simulink library "GTM_aerolib"  (Simulink 7.2)
settings: Solver=ode45  SolverMode=SingleTasking  StartTime=0.0  StopTime=10.0  RelTol=1e-3
undefined symbols (not defined in the file or in its folder): Aero, DamageModels
libraries: simulink_need_slupdate x58, GTM_aerolib x8, simulink x3
(part 2 of 3)

== system GTM_aerolib/Merged Control Surfaces/Spoilers ==
  alpha : Inport  OutDataType=sfix(16)  OutScaling=2^0
  beta : Inport  Port=2  OutDataType=sfix(16)  OutScaling=2^0
  Left : Inport  Port=3  OutDataType=sfix(16)  OutScaling=2^0
  Right : Inport  Port=4  OutDataType=sfix(16)  OutScaling=2^0
  Constant1 : Constant  Value=[0:5]  OutDataTypeMode=uint32  OutDataType=sfix(16)  OutScaling=2^0  OutDataTypeStr=uint32
  Constant2 : Constant  Value=[0:5]  OutDataTypeMode=uint32  OutDataType=sfix(16)  OutScaling=2^0  OutDataTypeStr=uint32
  Gain2 : Gain  Gain=-1  ParameterDataType=sfix(16)  ParameterScaling=2^0  OutDataType=sfix(16)  OutScaling=2^0
  Negate Lateral : Gain  Gain=[1 -1 1 -1 1 -1]  ParameterDataType=sfix(16)  ParameterScaling=2^0  OutDataType=sfix(16)  OutScaling=2^0
  PreLookup Index Search : simulink_need_slupdate/PreLookup Index Search  bpData=Aero.dC6_spo.alpha  searchMode=Binary Search  cacheBpFlag=on  outputFlag=off  IndexDataType=uint32  extrapMode=Linear Extrapolation  rangeErrorMode=None
  PreLookup Index Search1 : simulink_need_slupdate/PreLookup Index Search  bpData=Aero.dC6_spo.beta  searchMode=Binary Search  cacheBpFlag=on  outputFlag=off  IndexDataType=uint32  extrapMode=Linear Extrapolation  rangeErrorMode=None
  PreLookup Index Search2 : simulink_need_slupdate/PreLookup Index Search  bpData=Aero.dC6_spo.spo  searchMode=Binary Search  cacheBpFlag=on  outputFlag=off  IndexDataType=uint32  extrapMode=Linear Extrapolation  rangeErrorMode=None
  PreLookup Index Search3 : simulink_need_slupdate/PreLookup Index Search  bpData=Aero.dC6_spo.beta  searchMode=Binary Search  cacheBpFlag=on  outputFlag=off  IndexDataType=uint32  extrapMode=Linear Extrapolation  rangeErrorMode=None
  PreLookup Index Search4 : simulink_need_slupdate/PreLookup Index Search  bpData=Aero.dC6_spo.spo  searchMode=Binary Search  cacheBpFlag=on  outputFlag=off  IndexDataType=uint32  extrapMode=Linear Extrapolation  rangeErrorMode=None
  Sum : Sum  Inputs=+|+  OutDataType=sfix(16)  OutScaling=2^0
  TableLookup : simulink_need_slupdate/Interpolation (n-D) using PreLookup  numDimsPopupSelect=4  explicitNumDims=2  table=Aero.dC6_spo.data  interpMethod=Linear  extrapMethod=Linear  rangeErrorMode=None  NumSelectionDims=1
  TableLookup1 : simulink_need_slupdate/Interpolation (n-D) using PreLookup  numDimsPopupSelect=4  explicitNumDims=2  table=Aero.dC6_spo.data  interpMethod=Linear  extrapMethod=Linear  rangeErrorMode=None  NumSelectionDims=1
  dC6 : Outport  OutDataType=sfix(16)  OutScaling=2^0
  wires:
  Left/1 -> PreLookup Index Search2/1
  alpha/1 -> PreLookup Index Search/1
  beta/1 -> PreLookup Index Search3/1, Gain2/1
  Sum/1 -> dC6/1
  PreLookup Index Search/1 -> TableLookup/1, TableLookup1/1
  PreLookup Index Search1/1 -> TableLookup/2
  PreLookup Index Search2/1 -> TableLookup/3
  PreLookup Index Search3/1 -> TableLookup1/2
  TableLookup1/1 -> Sum/2
  TableLookup/1 -> Negate Lateral/1
  Right/1 -> PreLookup Index Search4/1
  PreLookup Index Search4/1 -> TableLookup1/3
  Constant2/1 -> TableLookup/4
  Constant1/1 -> TableLookup1/4
  Gain2/1 -> PreLookup Index Search1/1
  Negate Lateral/1 -> Sum/1

== system GTM_aerolib/Basic Airframe/DamageEffects/Switch Case Action Subsystem ==
  alpha : Inport  OutDataType=sfix(16)  OutScaling=2^0
  beta : Inport  Port=2  OutDataType=sfix(16)  OutScaling=2^0
  damage_case : Inport  Port=3  OutDataType=sfix(16)  OutScaling=2^0
  Action Port : ActionPort  ActionType=case
  AlphaLookup : PreLookup  BreakpointsData=Aero.dC6_damage.bas.alpha  BeginIndexSearchUsingPreviousIndexResult=on  ProcessOutOfRangeInput=Linear extrapolation  IndexDataType=sfix(16)  FractionDataType=sfix(16)  FractionScaling=2^0
  BetaLookup : PreLookup  BreakpointsData=Aero.dC6_damage.bas.beta  ProcessOutOfRangeInput=Linear extrapolation  IndexDataType=sfix(16)  FractionDataType=sfix(16)  FractionScaling=2^0
  Constant : Constant  Value=uint32(1)  OutDataType=sfix(16)  OutScaling=2^0
  Constant4 : Constant  Value=[0:5]  OutDataTypeMode=uint32  OutDataType=sfix(16)  OutScaling=2^0  OutDataTypeStr=uint32
  Interpolation Using Prelookup : Interpolation_n-D  NumberOfTableDimensions=4  Table=Aero.dC6_damage.bas.data  ExtrapMethod=None - Clip  NumSelectionDims=2  OutDataType=sfix(16)  OutScaling=2^0
  Subtract : Sum  Inputs=+-  OutDataType=sfix(16)  OutScaling=2^-10
  dC6_dam : Outport  OutDataType=sfix(16)  OutScaling=2^0  InitialOutput=zeros(6,1)
  wires:
  Constant4/1 -> Interpolation Using Prelookup/6
  alpha/1 -> AlphaLookup/1
  beta/1 -> BetaLookup/1
  Interpolation Using Prelookup/1 -> dC6_dam/1
  AlphaLookup/1 -> Interpolation Using Prelookup/1
  AlphaLookup/2 -> Interpolation Using Prelookup/2
  BetaLookup/1 -> Interpolation Using Prelookup/3
  BetaLookup/2 -> Interpolation Using Prelookup/4
  damage_case/1 -> Subtract/1
  Subtract/1 -> Interpolation Using Prelookup/5
  Constant/1 -> Subtract/2

== system GTM_aerolib/Basic Airframe/DamageEffects/Switch Case Action Subsystem2 ==
  Action Port : ActionPort  ActionType=default
  Constant4 : Constant  Value=zeros(6,1)  OutDataTypeMode=double  OutDataType=sfix(16)  OutScaling=2^0  OutDataTypeStr=double
  Zeros : Outport  OutDataType=sfix(16)  OutScaling=2^0  InitialOutput=zeros(6,1)
  wires:
  Constant4/1 -> Zeros/1

== system GTM_aerolib/Control Surfaces/Elevator/Stab1/Stab/Elev Table ==
  alpha_k : Inport  OutDataType=sfix(16)  OutScaling=2^0
  alpha_f : Inport  Port=2  OutDataType=sfix(16)  OutScaling=2^0
  beta_k : Inport  Port=3  OutDataType=sfix(16)  OutScaling=2^0
  beta_f : Inport  Port=4  OutDataType=sfix(16)  OutScaling=2^0
  stab_k : Inport  Port=5  OutDataType=sfix(16)  OutScaling=2^0
  stab_f : Inport  Port=6  OutDataType=sfix(16)  OutScaling=2^0
  elev : Inport  Port=7  OutDataType=sfix(16)  OutScaling=2^0
  Assignment to  Longitudinal : Assignment  IndexMode=Zero-based  IndexOptions=Index vector (dialog)  Indices=[0 2 4]  OutputSizes=[1 1]
  Constant : Constant  Value=zeros(6,1)  OutDataType=sfix(16)  OutScaling=2^0
  Constant2 : Constant  Value=[0:2]  OutDataTypeMode=uint32  OutDataType=sfix(16)  OutScaling=2^0  OutDataTypeStr=uint32
  Interpolation Using Prelookup : Interpolation_n-D  NumberOfTableDimensions=5  Table=Aero.dC3_ele.data  NumSelectionDims=1  OutDataType=sfix(16)  OutScaling=2^0
  Prelookup4 : PreLookup  BreakpointsData=Aero.dC3_ele.elev  IndexSearchMethod=Linear search  BeginIndexSearchUsingPreviousIndexResult=on  ProcessOutOfRangeInput=Linear extrapolation  IndexDataType=sfix(16)  FractionDataType=sfix(16)  FractionScaling=2^0
  dC6 : Outport  OutDataType=sfix(16)  OutScaling=2^0
  wires:
  Assignment to  Longitudinal/1 -> dC6/1
  Interpolation Using Prelookup/1 -> Assignment to  Longitudinal/2
  Constant/1 -> Assignment to  Longitudinal/1
  elev/1 -> Prelookup4/1
  stab_k/1 -> Interpolation Using Prelookup/5
  beta_k/1 -> Interpolation Using Prelookup/3
  alpha_k/1 -> Interpolation Using Prelookup/1
  alpha_f/1 -> Interpolation Using Prelookup/2
  beta_f/1 -> Interpolation Using Prelookup/4
  stab_f/1 -> Interpolation Using Prelookup/6
  Prelookup4/1 -> Interpolation Using Prelookup/7
  Prelookup4/2 -> Interpolation Using Prelookup/8
  Constant2/1 -> Interpolation Using Prelookup/9

== system GTM_aerolib/Control Surfaces/Elevator/Stab1/Stab/Elev Table0 ==
  alpha_k : Inport  OutDataType=sfix(16)  OutScaling=2^0
  alpha_f : Inport  Port=2  OutDataType=sfix(16)  OutScaling=2^0
  beta_k : Inport  Port=3  OutDataType=sfix(16)  OutScaling=2^0
  beta_f : Inport  Port=4  OutDataType=sfix(16)  OutScaling=2^0
  stab_k : Inport  Port=5  OutDataType=sfix(16)  OutScaling=2^0
  stab_f : Inport  Port=6  OutDataType=sfix(16)  OutScaling=2^0
  elev : Inport  Port=7  OutDataType=sfix(16)  OutScaling=2^0
  Assignment to  Longitudinal : Assignment  IndexMode=Zero-based  IndexOptions=Index vector (dialog)  Indices=[0 2 4]  OutputSizes=[1 1]
  Constant : Constant  Value=zeros(6,1)  OutDataType=sfix(16)  OutScaling=2^0
  Constant2 : Constant  Value=[0:2]  OutDataTypeMode=uint32  OutDataType=sfix(16)  OutScaling=2^0  OutDataTypeStr=uint32
  Interpolation Using Prelookup : Interpolation_n-D  NumberOfTableDimensions=5  Table=Aero.dC3_ele.data  NumSelectionDims=1  OutDataType=sfix(16)  OutScaling=2^0
  Prelookup4 : PreLookup  BreakpointsData=Aero.dC3_ele.elev  IndexSearchMethod=Linear search  BeginIndexSearchUsingPreviousIndexResult=on  ProcessOutOfRangeInput=Linear extrapolation  IndexDataType=sfix(16)  FractionDataType=sfix(16)  FractionScaling=2^0
  dC6 : Outport  OutDataType=sfix(16)  OutScaling=2^0
  wires:
  Assignment to  Longitudinal/1 -> dC6/1
  Interpolation Using Prelookup/1 -> Assignment to  Longitudinal/2
  Constant/1 -> Assignment to  Longitudinal/1
  elev/1 -> Prelookup4/1
  stab_k/1 -> Interpolation Using Prelookup/5
  beta_k/1 -> Interpolation Using Prelookup/3
  alpha_k/1 -> Interpolation Using Prelookup/1
  alpha_f/1 -> Interpolation Using Prelookup/2
  beta_f/1 -> Interpolation Using Prelookup/4
  stab_f/1 -> Interpolation Using Prelookup/6
  Prelookup4/1 -> Interpolation Using Prelookup/7
  Prelookup4/2 -> Interpolation Using Prelookup/8
  Constant2/1 -> Interpolation Using Prelookup/9

== system GTM_aerolib/Control Surfaces/Elevator/Stab1/Stab/Elev Table1 ==
  alpha_k : Inport  OutDataType=sfix(16)  OutScaling=2^0
  alpha_f : Inport  Port=2  OutDataType=sfix(16)  OutScaling=2^0
  beta_k : Inport  Port=3  OutDataType=sfix(16)  OutScaling=2^0
  beta_f : Inport  Port=4  OutDataType=sfix(16)  OutScaling=2^0
  stab_k : Inport  Port=5  OutDataType=sfix(16)  OutScaling=2^0
  stab_f : Inport  Port=6  OutDataType=sfix(16)  OutScaling=2^0
  elev : Inport  Port=7  OutDataType=sfix(16)  OutScaling=2^0
  Assignment to  Longitudinal : Assignment  IndexMode=Zero-based  IndexOptions=Index vector (dialog)  Indices=[0 2 4]  OutputSizes=[1 1]
  Constant : Constant  Value=zeros(6,1)  OutDataType=sfix(16)  OutScaling=2^0
  Constant2 : Constant  Value=[0:2]  OutDataTypeMode=uint32  OutDataType=sfix(16)  OutScaling=2^0  OutDataTypeStr=uint32
  Interpolation Using Prelookup : Interpolation_n-D  NumberOfTableDimensions=5  Table=Aero.dC3_ele.data  NumSelectionDims=1  OutDataType=sfix(16)  OutScaling=2^0
  Prelookup4 : PreLookup  BreakpointsData=Aero.dC3_ele.elev  IndexSearchMethod=Linear search  BeginIndexSearchUsingPreviousIndexResult=on  ProcessOutOfRangeInput=Linear extrapolation  IndexDataType=sfix(16)  FractionDataType=sfix(16)  FractionScaling=2^0
  dC6 : Outport  OutDataType=sfix(16)  OutScaling=2^0
  wires:
  Assignment to  Longitudinal/1 -> dC6/1
  Interpolation Using Prelookup/1 -> Assignment to  Longitudinal/2
  Constant/1 -> Assignment to  Longitudinal/1
  elev/1 -> Prelookup4/1
  stab_k/1 -> Interpolation Using Prelookup/5
  beta_k/1 -> Interpolation Using Prelookup/3
  alpha_k/1 -> Interpolation Using Prelookup/1
  alpha_f/1 -> Interpolation Using Prelookup/2
  beta_f/1 -> Interpolation Using Prelookup/4
  stab_f/1 -> Interpolation Using Prelookup/6
  Prelookup4/1 -> Interpolation Using Prelookup/7
  Prelookup4/2 -> Interpolation Using Prelookup/8
  Constant2/1 -> Interpolation Using Prelookup/9

== system GTM_aerolib/Control Surfaces/Elevator/Stab1/Stab/Elev Table2 ==
  alpha_k : Inport  OutDataType=sfix(16)  OutScaling=2^0
  alpha_f : Inport  Port=2  OutDataType=sfix(16)  OutScaling=2^0
  beta_k : Inport  Port=3  OutDataType=sfix(16)  OutScaling=2^0
  beta_f : Inport  Port=4  OutDataType=sfix(16)  OutScaling=2^0
  stab_k : Inport  Port=5  OutDataType=sfix(16)  OutScaling=2^0
  stab_f : Inport  Port=6  OutDataType=sfix(16)  OutScaling=2^0
  elev : Inport  Port=7  OutDataType=sfix(16)  OutScaling=2^0
  Assignment to  Longitudinal : Assignment  IndexMode=Zero-based  IndexOptions=Index vector (dialog)  Indices=[0 2 4]  OutputSizes=[1 1]
  Constant : Constant  Value=zeros(6,1)  OutDataType=sfix(16)  OutScaling=2^0
  Constant2 : Constant  Value=[0:2]  OutDataTypeMode=uint32  OutDataType=sfix(16)  OutScaling=2^0  OutDataTypeStr=uint32
  Interpolation Using Prelookup : Interpolation_n-D  NumberOfTableDimensions=5  Table=Aero.dC3_ele.data  NumSelectionDims=1  OutDataType=sfix(16)  OutScaling=2^0
  Prelookup4 : PreLookup  BreakpointsData=Aero.dC3_ele.elev  IndexSearchMethod=Linear search  BeginIndexSearchUsingPreviousIndexResult=on  ProcessOutOfRangeInput=Linear extrapolation  IndexDataType=sfix(16)  FractionDataType=sfix(16)  FractionScaling=2^0
  dC6 : Outport  OutDataType=sfix(16)  OutScaling=2^0
  wires:
  Assignment to  Longitudinal/1 -> dC6/1
  Interpolation Using Prelookup/1 -> Assignment to  Longitudinal/2
  Constant/1 -> Assignment to  Longitudinal/1
  elev/1 -> Prelookup4/1
  stab_k/1 -> Interpolation Using Prelookup/5
  beta_k/1 -> Interpolation Using Prelookup/3
  alpha_k/1 -> Interpolation Using Prelookup/1
  alpha_f/1 -> Interpolation Using Prelookup/2
  beta_f/1 -> Interpolation Using Prelookup/4
  stab_f/1 -> Interpolation Using Prelookup/6
  Prelookup4/1 -> Interpolation Using Prelookup/7
  Prelookup4/2 -> Interpolation Using Prelookup/8
  Constant2/1 -> Interpolation Using Prelookup/9

== system GTM_aerolib/Control Surfaces/Elevator/Stab1/Stab/Elev Table3 ==
  alpha_k : Inport  OutDataType=sfix(16)  OutScaling=2^0
  alpha_f : Inport  Port=2  OutDataType=sfix(16)  OutScaling=2^0
  beta_k : Inport  Port=3  OutDataType=sfix(16)  OutScaling=2^0
  beta_f : Inport  Port=4  OutDataType=sfix(16)  OutScaling=2^0
  stab_k : Inport  Port=5  OutDataType=sfix(16)  OutScaling=2^0
  stab_f : Inport  Port=6  OutDataType=sfix(16)  OutScaling=2^0
  elev : Inport  Port=7  OutDataType=sfix(16)  OutScaling=2^0
  Assignment to  Longitudinal : Assignment  IndexMode=Zero-based  IndexOptions=Index vector (dialog)  Indices=[0 2 4]  OutputSizes=[1 1]
  Constant : Constant  Value=zeros(6,1)  OutDataType=sfix(16)  OutScaling=2^0
  Constant2 : Constant  Value=[0:2]  OutDataTypeMode=uint32  OutDataType=sfix(16)  OutScaling=2^0  OutDataTypeStr=uint32
  Interpolation Using Prelookup : Interpolation_n-D  NumberOfTableDimensions=5  Table=Aero.dC3_ele.data  NumSelectionDims=1  OutDataType=sfix(16)  OutScaling=2^0
  Prelookup4 : PreLookup  BreakpointsData=Aero.dC3_ele.elev  IndexSearchMethod=Linear search  BeginIndexSearchUsingPreviousIndexResult=on  ProcessOutOfRangeInput=Linear extrapolation  IndexDataType=sfix(16)  FractionDataType=sfix(16)  FractionScaling=2^0
  dC6 : Outport  OutDataType=sfix(16)  OutScaling=2^0
  wires:
  Assignment to  Longitudinal/1 -> dC6/1
  Interpolation Using Prelookup/1 -> Assignment to  Longitudinal/2
  Constant/1 -> Assignment to  Longitudinal/1
  elev/1 -> Prelookup4/1
  stab_k/1 -> Interpolation Using Prelookup/5
  beta_k/1 -> Interpolation Using Prelookup/3
  alpha_k/1 -> Interpolation Using Prelookup/1
  alpha_f/1 -> Interpolation Using Prelookup/2
  beta_f/1 -> Interpolation Using Prelookup/4
  stab_f/1 -> Interpolation Using Prelookup/6
  Prelookup4/1 -> Interpolation Using Prelookup/7
  Prelookup4/2 -> Interpolation Using Prelookup/8
  Constant2/1 -> Interpolation Using Prelookup/9

== system GTM_aerolib/Control Surfaces/Flaps/Flap Table ==
  alpha_k : Inport  OutDataType=sfix(16)  OutScaling=2^0
  alpha_f : Inport  Port=2  OutDataType=sfix(16)  OutScaling=2^0
  flap : Inport  Port=3  OutDataType=sfix(16)  OutScaling=2^0
  Assignment to  Longitudinal : Assignment  IndexMode=Zero-based  IndexOptions=Index vector (dialog)  Indices=[0 2 4]  OutputSizes=[1 1]
  Constant : Constant  Value=zeros(6,1)  OutDataType=sfix(16)  OutScaling=2^0
  Constant2 : Constant  Value=[0:2]  OutDataTypeMode=uint32  OutDataType=sfix(16)  OutScaling=2^0  OutDataTypeStr=uint32
  Interpolation Using Prelookup : Interpolation_n-D  NumberOfTableDimensions=3  Table=Aero.dC3_flp.data  NumSelectionDims=1  OutDataType=sfix(16)  OutScaling=2^0
  Prelookup1 : PreLookup  BreakpointsData=Aero.dC3_flp.flap  IndexSearchMethod=Linear search  BeginIndexSearchUsingPreviousIndexResult=on  ProcessOutOfRangeInput=Linear extrapolation  IndexDataType=sfix(16)  FractionDataType=sfix(16)  FractionScaling=2^0
  dC6 : Outport  OutDataType=sfix(16)  OutScaling=2^0
  wires:
  Assignment to  Longitudinal/1 -> dC6/1
  Constant/1 -> Assignment to  Longitudinal/1
  flap/1 -> Prelookup1/1
  alpha_k/1 -> Interpolation Using Prelookup/1
  alpha_f/1 -> Interpolation Using Prelookup/2
  Constant2/1 -> Interpolation Using Prelookup/5
  Prelookup1/1 -> Interpolation Using Prelookup/3
  Prelookup1/2 -> Interpolation Using Prelookup/4
  Interpolation Using Prelookup/1 -> Assignment to  Longitudinal/2

== system GTM_aerolib/Control Surfaces/Flaps/Flap Table1 ==
  alpha_k : Inport  OutDataType=sfix(16)  OutScaling=2^0
  alpha_f : Inport  Port=2  OutDataType=sfix(16)  OutScaling=2^0
  flap : Inport  Port=3  OutDataType=sfix(16)  OutScaling=2^0
  Assignment to  Longitudinal : Assignment  IndexMode=Zero-based  IndexOptions=Index vector (dialog)  Indices=[0 2 4]  OutputSizes=[1 1]
  Constant : Constant  Value=zeros(6,1)  OutDataType=sfix(16)  OutScaling=2^0
  Constant2 : Constant  Value=[0:2]  OutDataTypeMode=uint32  OutDataType=sfix(16)  OutScaling=2^0  OutDataTypeStr=uint32
  Interpolation Using Prelookup : Interpolation_n-D  NumberOfTableDimensions=3  Table=Aero.dC3_flp.data  NumSelectionDims=1  OutDataType=sfix(16)  OutScaling=2^0
  Prelookup1 : PreLookup  BreakpointsData=Aero.dC3_flp.flap  IndexSearchMethod=Linear search  BeginIndexSearchUsingPreviousIndexResult=on  ProcessOutOfRangeInput=Linear extrapolation  IndexDataType=sfix(16)  FractionDataType=sfix(16)  FractionScaling=2^0
  dC6 : Outport  OutDataType=sfix(16)  OutScaling=2^0
  wires:
  Interpolation Using Prelookup/1 -> Assignment to  Longitudinal/2
  Prelookup1/2 -> Interpolation Using Prelookup/4
  Prelookup1/1 -> Interpolation Using Prelookup/3
  Constant2/1 -> Interpolation Using Prelookup/5
  alpha_f/1 -> Interpolation Using Prelookup/2
  alpha_k/1 -> Interpolation Using Prelookup/1
  flap/1 -> Prelookup1/1
  Constant/1 -> Assignment to  Longitudinal/1
  Assignment to  Longitudinal/1 -> dC6/1

== system GTM_aerolib/Control Surfaces/Flaps/Flap Table2 ==
  alpha_k : Inport  OutDataType=sfix(16)  OutScaling=2^0
  alpha_f : Inport  Port=2  OutDataType=sfix(16)  OutScaling=2^0
  flap : Inport  Port=3  OutDataType=sfix(16)  OutScaling=2^0
  Assignment to  Longitudinal : Assignment  IndexMode=Zero-based  IndexOptions=Index vector (dialog)  Indices=[0 2 4]  OutputSizes=[1 1]
  Constant : Constant  Value=zeros(6,1)  OutDataType=sfix(16)  OutScaling=2^0
  Constant2 : Constant  Value=[0:2]  OutDataTypeMode=uint32  OutDataType=sfix(16)  OutScaling=2^0  OutDataTypeStr=uint32
  Interpolation Using Prelookup : Interpolation_n-D  NumberOfTableDimensions=3  Table=Aero.dC3_flp.data  NumSelectionDims=1  OutDataType=sfix(16)  OutScaling=2^0
  Prelookup1 : PreLookup  BreakpointsData=Aero.dC3_flp.flap  IndexSearchMethod=Linear search  BeginIndexSearchUsingPreviousIndexResult=on  ProcessOutOfRangeInput=Linear extrapolation  IndexDataType=sfix(16)  FractionDataType=sfix(16)  FractionScaling=2^0
  dC6 : Outport  OutDataType=sfix(16)  OutScaling=2^0
  wires:
  Interpolation Using Prelookup/1 -> Assignment to  Longitudinal/2
  Prelookup1/2 -> Interpolation Using Prelookup/4
  Prelookup1/1 -> Interpolation Using Prelookup/3
  Constant2/1 -> Interpolation Using Prelookup/5
  alpha_f/1 -> Interpolation Using Prelookup/2
  alpha_k/1 -> Interpolation Using Prelookup/1
  flap/1 -> Prelookup1/1
  Constant/1 -> Assignment to  Longitudinal/1
  Assignment to  Longitudinal/1 -> dC6/1

== system GTM_aerolib/Control Surfaces/Flaps/Flap Table3 ==
  alpha_k : Inport  OutDataType=sfix(16)  OutScaling=2^0
  alpha_f : Inport  Port=2  OutDataType=sfix(16)  OutScaling=2^0
  flap : Inport  Port=3  OutDataType=sfix(16)  OutScaling=2^0
  Assignment to  Longitudinal : Assignment  IndexMode=Zero-based  IndexOptions=Index vector (dialog)  Indices=[0 2 4]  OutputSizes=[1 1]
  Constant : Constant  Value=zeros(6,1)  OutDataType=sfix(16)  OutScaling=2^0
  Constant2 : Constant  Value=[0:2]  OutDataTypeMode=uint32  OutDataType=sfix(16)  OutScaling=2^0  OutDataTypeStr=uint32
  Interpolation Using Prelookup : Interpolation_n-D  NumberOfTableDimensions=3  Table=Aero.dC3_flp.data  NumSelectionDims=1  OutDataType=sfix(16)  OutScaling=2^0
  Prelookup1 : PreLookup  BreakpointsData=Aero.dC3_flp.flap  IndexSearchMethod=Linear search  BeginIndexSearchUsingPreviousIndexResult=on  ProcessOutOfRangeInput=Linear extrapolation  IndexDataType=sfix(16)  FractionDataType=sfix(16)  FractionScaling=2^0
  dC6 : Outport  OutDataType=sfix(16)  OutScaling=2^0
  wires:
  Interpolation Using Prelookup/1 -> Assignment to  Longitudinal/2
  Prelookup1/2 -> Interpolation Using Prelookup/4
  Prelookup1/1 -> Interpolation Using Prelookup/3
  Constant2/1 -> Interpolation Using Prelookup/5
  alpha_f/1 -> Interpolation Using Prelookup/2
  alpha_k/1 -> Interpolation Using Prelookup/1
  flap/1 -> Prelookup1/1
  Constant/1 -> Assignment to  Longitudinal/1
  Assignment to  Longitudinal/1 -> dC6/1

== system GTM_aerolib/Control Surfaces/Rudder/Gains ==
  dC6_in : Inport  OutDataType=sfix(16)  OutScaling=2^0
  Product : Product  OutDataType=sfix(16)  OutScaling=2^0  RndMeth=Zero
  gains : Constant  Value=gains  OutDataType=sfix(16)  OutScaling=2^0
  dC6 : Outport  OutDataType=sfix(16)  OutScaling=2^0
  wires:
  gains/1 -> Product/2
  Product/1 -> dC6/1
  dC6_in/1 -> Product/1

== system GTM_aerolib/Control Surfaces/Rudder/Gains1 ==
  dC6_in : Inport  OutDataType=sfix(16)  OutScaling=2^0
  Product : Product  OutDataType=sfix(16)  OutScaling=2^0  RndMeth=Zero
  gains : Constant  Value=gains  OutDataType=sfix(16)  OutScaling=2^0
  dC6 : Outport  OutDataType=sfix(16)  OutScaling=2^0
  wires:
  dC6_in/1 -> Product/1
  Product/1 -> dC6/1
  gains/1 -> Product/2

== system GTM_aerolib/Control Surfaces/Rudder/Lower Rudder ==
  alpha : Inport  OutDataType=sfix(16)  OutScaling=2^0
  beta : Inport  Port=2  OutDataType=sfix(16)  OutScaling=2^0
  rud : Inport  Port=3  OutDataType=sfix(16)  OutScaling=2^0
  Abs : Abs
  Assignment to lateral : Assignment  IndexMode=Zero-based  IndexOptions=Index vector (dialog)  Indices=[1 3 5]  OutputSizes=[1 1]
  Constant : Constant  Value=-1  OutDataType=sfix(16)  OutScaling=2^0
  Constant1 : Constant  OutDataType=sfix(16)  OutScaling=2^0
  Constant2 : Constant  Value=[0:5]  OutDataTypeMode=uint32  OutDataType=sfix(16)  OutScaling=2^0  OutDataTypeStr=uint32
  Constant3 : Constant  Value=ones(6,1)  OutDataType=sfix(16)  OutScaling=2^0
  Gain : Gain  Gain=-1  ParameterDataType=sfix(16)  ParameterScaling=2^0  OutDataType=sfix(16)  OutScaling=2^0
  Interpolation Using Prelookup : Interpolation_n-D  NumberOfTableDimensions=4  Table=Aero.dC6_rud.data  NumSelectionDims=1  OutDataType=sfix(16)  OutScaling=2^0
  Prelookup : PreLookup  BreakpointsData=Aero.dC6_rud.alpha  IndexSearchMethod=Linear search  BeginIndexSearchUsingPreviousIndexResult=on  ProcessOutOfRangeInput=Linear extrapolation  IndexDataType=sfix(16)  FractionDataType=sfix(16)  FractionScaling=2^0
  Prelookup1 : PreLookup  BreakpointsData=Aero.dC6_rud.beta  IndexSearchMethod=Linear search  BeginIndexSearchUsingPreviousIndexResult=on  ProcessOutOfRangeInput=Linear extrapolation  IndexDataType=sfix(16)  FractionDataType=sfix(16)  FractionScaling=2^0
  Prelookup2 : PreLookup  BreakpointsData=Aero.dC6_rud.rud  IndexSearchMethod=Linear search  BeginIndexSearchUsingPreviousIndexResult=on  ProcessOutOfRangeInput=Linear extrapolation  IndexDataType=sfix(16)  FractionDataType=sfix(16)  FractionScaling=2^0
  Product1 : Product  OutDataType=sfix(16)  OutScaling=2^0  RndMeth=Zero
  Product2 : Product  OutDataType=sfix(16)  OutScaling=2^0  RndMeth=Zero
  Switch : Switch
  dC6 : Outport  OutDataType=sfix(16)  OutScaling=2^0
  wires:
  Constant2/1 -> Interpolation Using Prelookup/7
  Prelookup2/2 -> Interpolation Using Prelookup/6
  Prelookup2/1 -> Interpolation Using Prelookup/5
  Prelookup1/2 -> Interpolation Using Prelookup/4
  Prelookup1/1 -> Interpolation Using Prelookup/3
  Prelookup/2 -> Interpolation Using Prelookup/2
  Prelookup/1 -> Interpolation Using Prelookup/1
  Product1/1 -> Prelookup1/1
  rud/1 -> Abs/1, Switch/2
  Abs/1 -> Gain/1
  Gain/1 -> Prelookup2/1
  alpha/1 -> Prelookup/1
  beta/1 -> Product1/1
  Product2/1 -> dC6/1
  Constant/1 -> Switch/1
  Constant1/1 -> Switch/3
  Switch/1 -> Product1/2, Assignment to lateral/2
  Constant3/1 -> Assignment to lateral/1
  Assignment to lateral/1 -> Product2/2
  Interpolation Using Prelookup/1 -> Product2/1

== system GTM_aerolib/Control Surfaces/Rudder/Upper Rudder ==
  alpha : Inport  OutDataType=sfix(16)  OutScaling=2^0
  beta : Inport  Port=2  OutDataType=sfix(16)  OutScaling=2^0
  rud : Inport  Port=3  OutDataType=sfix(16)  OutScaling=2^0
  Abs : Abs
  Assignment to lateral : Assignment  IndexMode=Zero-based  IndexOptions=Index vector (dialog)  Indices=[1 3 5]  OutputSizes=[1 1]
  Constant : Constant  Value=-1  OutDataType=sfix(16)  OutScaling=2^0
  Constant1 : Constant  OutDataType=sfix(16)  OutScaling=2^0
  Constant2 : Constant  Value=[0:5]  OutDataTypeMode=uint32  OutDataType=sfix(16)  OutScaling=2^0  OutDataTypeStr=uint32
  Constant3 : Constant  Value=ones(6,1)  OutDataType=sfix(16)  OutScaling=2^0
  Gain : Gain  Gain=-1  ParameterDataType=sfix(16)  ParameterScaling=2^0  OutDataType=sfix(16)  OutScaling=2^0
  Interpolation Using Prelookup : Interpolation_n-D  NumberOfTableDimensions=4  Table=Aero.dC6_rud.data  NumSelectionDims=1  OutDataType=sfix(16)  OutScaling=2^0
  Prelookup : PreLookup  BreakpointsData=Aero.dC6_rud.alpha  IndexSearchMethod=Linear search  BeginIndexSearchUsingPreviousIndexResult=on  ProcessOutOfRangeInput=Linear extrapolation  IndexDataType=sfix(16)  FractionDataType=sfix(16)  FractionScaling=2^0
  Prelookup1 : PreLookup  BreakpointsData=Aero.dC6_rud.beta  IndexSearchMethod=Linear search  BeginIndexSearchUsingPreviousIndexResult=on  ProcessOutOfRangeInput=Linear extrapolation  IndexDataType=sfix(16)  FractionDataType=sfix(16)  FractionScaling=2^0
  Prelookup2 : PreLookup  BreakpointsData=Aero.dC6_rud.rud  IndexSearchMethod=Linear search  BeginIndexSearchUsingPreviousIndexResult=on  ProcessOutOfRangeInput=Linear extrapolation  IndexDataType=sfix(16)  FractionDataType=sfix(16)  FractionScaling=2^0
  Product1 : Product  OutDataType=sfix(16)  OutScaling=2^0  RndMeth=Zero
  Product2 : Product  OutDataType=sfix(16)  OutScaling=2^0  RndMeth=Zero
  Switch : Switch
  dC6 : Outport  OutDataType=sfix(16)  OutScaling=2^0
  wires:
  Interpolation Using Prelookup/1 -> Product2/1
  Assignment to lateral/1 -> Product2/2
  Constant3/1 -> Assignment to lateral/1
  Switch/1 -> Assignment to lateral/2, Product1/2
  Constant1/1 -> Switch/3
  Constant/1 -> Switch/1
  Product2/1 -> dC6/1
  beta/1 -> Product1/1
  alpha/1 -> Prelookup/1
  Gain/1 -> Prelookup2/1
  Abs/1 -> Gain/1
  rud/1 -> Switch/2, Abs/1
  Product1/1 -> Prelookup1/1
  Prelookup/1 -> Interpolation Using Prelookup/1
  Prelookup/2 -> Interpolation Using Prelookup/2
  Prelookup1/1 -> Interpolation Using Prelookup/3
  Prelookup1/2 -> Interpolation Using Prelookup/4
  Prelookup2/1 -> Interpolation Using Prelookup/5
  Prelookup2/2 -> Interpolation Using Prelookup/6
  Constant2/1 -> Interpolation Using Prelookup/7

== system GTM_aerolib/Control Surfaces/Spoilers/Gains1 ==
  dC6_in : Inport  OutDataType=sfix(16)  OutScaling=2^0
  Product : Product  OutDataType=sfix(16)  OutScaling=2^0  RndMeth=Zero
  gains : Constant  Value=gains  OutDataType=sfix(16)  OutScaling=2^0
  dC6 : Outport  OutDataType=sfix(16)  OutScaling=2^0
  wires:
  gains/1 -> Product/2
  Product/1 -> dC6/1
  dC6_in/1 -> Product/1

== system GTM_aerolib/Control Surfaces/Spoilers/Gains2 ==
  dC6_in : Inport  OutDataType=sfix(16)  OutScaling=2^0
  Product : Product  OutDataType=sfix(16)  OutScaling=2^0  RndMeth=Zero
  gains : Constant  Value=gains  OutDataType=sfix(16)  OutScaling=2^0
  dC6 : Outport  OutDataType=sfix(16)  OutScaling=2^0
  wires:
  dC6_in/1 -> Product/1
  Product/1 -> dC6/1
  gains/1 -> Product/2

== system GTM_aerolib/Control Surfaces/Spoilers/Gains3 ==
  dC6_in : Inport  OutDataType=sfix(16)  OutScaling=2^0
  Product : Product  OutDataType=sfix(16)  OutScaling=2^0  RndMeth=Zero
  gains : Constant  Value=gains  OutDataType=sfix(16)  OutScaling=2^0
  dC6 : Outport  OutDataType=sfix(16)  OutScaling=2^0
  wires:
  dC6_in/1 -> Product/1
  Product/1 -> dC6/1
  gains/1 -> Product/2

== system GTM_aerolib/Control Surfaces/Spoilers/Gains4 ==
  dC6_in : Inport  OutDataType=sfix(16)  OutScaling=2^0
  Product : Product  OutDataType=sfix(16)  OutScaling=2^0  RndMeth=Zero
  gains : Constant  Value=gains  OutDataType=sfix(16)  OutScaling=2^0
  dC6 : Outport  OutDataType=sfix(16)  OutScaling=2^0
  wires:
  gains/1 -> Product/2
  Product/1 -> dC6/1
  dC6_in/1 -> Product/1

== system GTM_aerolib/Control Surfaces/Spoilers/InboardSpoilers ==
  alpha : Inport  OutDataType=sfix(16)  OutScaling=2^0
  beta : Inport  Port=2  OutDataType=sfix(16)  OutScaling=2^0
  SPLLIB : Inport  Port=3  OutDataType=sfix(16)  OutScaling=2^0
  SPLRIB : Inport  Port=4  OutDataType=sfix(16)  OutScaling=2^0
  Constant1 : Constant  Value=[0:5]  OutDataTypeMode=uint32  OutDataType=sfix(16)  OutScaling=2^0  OutDataTypeStr=uint32
  Constant3 : Constant  Value=[0:5]  OutDataTypeMode=uint32  OutDataType=sfix(16)  OutScaling=2^0  OutDataTypeStr=uint32
  Gain2 : Gain  Gain=-1  ParameterDataType=sfix(16)  ParameterScaling=2^0  OutDataType=sfix(16)  OutScaling=2^0
  Interpolation Using Prelookup : Interpolation_n-D  NumberOfTableDimensions=4  Table=Aero.dC6_spo.data  NumSelectionDims=1  OutDataType=sfix(16)  OutScaling=2^0
  Interpolation Using Prelookup1 : Interpolation_n-D  NumberOfTableDimensions=4  Table=Aero.dC6_spo.data  NumSelectionDims=1  OutDataType=sfix(16)  OutScaling=2^0
  Negate Lateral : Gain  Gain=[1 -1 1 -1 1 -1]  ParameterDataType=sfix(16)  ParameterScaling=2^0  OutDataType=sfix(16)  OutScaling=2^0
  Prelookup1 : PreLookup  BreakpointsData=Aero.dC6_spo.alpha  IndexSearchMethod=Linear search  BeginIndexSearchUsingPreviousIndexResult=on  ProcessOutOfRangeInput=Linear extrapolation  IndexDataType=sfix(16)  FractionDataType=sfix(16)  FractionScaling=2^0
  Prelookup2 : PreLookup  BreakpointsData=Aero.dC6_spo.beta  IndexSearchMethod=Linear search  BeginIndexSearchUsingPreviousIndexResult=on  ProcessOutOfRangeInput=Linear extrapolation  IndexDataType=sfix(16)  FractionDataType=sfix(16)  FractionScaling=2^0
  Prelookup3 : PreLookup  BreakpointsData=Aero.dC6_spo.spo  IndexSearchMethod=Linear search  BeginIndexSearchUsingPreviousIndexResult=on  ProcessOutOfRangeInput=Linear extrapolation  IndexDataType=sfix(16)  FractionDataType=sfix(16)  FractionScaling=2^0
  Prelookup4 : PreLookup  BreakpointsData=Aero.dC6_spo.beta  IndexSearchMethod=Linear search  BeginIndexSearchUsingPreviousIndexResult=on  ProcessOutOfRangeInput=Linear extrapolation  IndexDataType=sfix(16)  FractionDataType=sfix(16)  FractionScaling=2^0
  Prelookup5 : PreLookup  BreakpointsData=Aero.dC6_spo.spo  IndexSearchMethod=Linear search  BeginIndexSearchUsingPreviousIndexResult=on  ProcessOutOfRangeInput=Linear extrapolation  IndexDataType=sfix(16)  FractionDataType=sfix(16)  FractionScaling=2^0
  Left : Outport  OutDataType=sfix(16)  OutScaling=2^0
  Right : Outport  Port=2  OutDataType=sfix(16)  OutScaling=2^0
  wires:
  Interpolation Using Prelookup/1 -> Negate Lateral/1
  Constant1/1 -> Interpolation Using Prelookup1/7
  Prelookup5/2 -> Interpolation Using Prelookup1/6
  Prelookup5/1 -> Interpolation Using Prelookup1/5
  Prelookup4/2 -> Interpolation Using Prelookup1/4
  Prelookup4/1 -> Interpolation Using Prelookup1/3
  Constant3/1 -> Interpolation Using Prelookup/7
  Prelookup3/2 -> Interpolation Using Prelookup/6
  Prelookup3/1 -> Interpolation Using Prelookup/5
  Prelookup2/2 -> Interpolation Using Prelookup/4
  Prelookup2/1 -> Interpolation Using Prelookup/3
  Prelookup1/2 -> Interpolation Using Prelookup1/2, Interpolation Using Prelookup/2
  Prelookup1/1 -> Interpolation Using Prelookup1/1, Interpolation Using Prelookup/1
  SPLLIB/1 -> Prelookup3/1
  alpha/1 -> Prelookup1/1
  beta/1 -> Prelookup4/1, Gain2/1
  SPLRIB/1 -> Prelookup5/1
  Interpolation Using Prelookup1/1 -> Right/1
  Negate Lateral/1 -> Left/1
  Gain2/1 -> Prelookup2/1

== system GTM_aerolib/Control Surfaces/Spoilers/OutboardSpoilers ==
  alpha : Inport  OutDataType=sfix(16)  OutScaling=2^0
  beta : Inport  Port=2  OutDataType=sfix(16)  OutScaling=2^0
  SPLLIB : Inport  Port=3  OutDataType=sfix(16)  OutScaling=2^0
  SPLRIB : Inport  Port=4  OutDataType=sfix(16)  OutScaling=2^0
  Constant1 : Constant  Value=[0:5]  OutDataTypeMode=uint32  OutDataType=sfix(16)  OutScaling=2^0  OutDataTypeStr=uint32
  Constant3 : Constant  Value=[0:5]  OutDataTypeMode=uint32  OutDataType=sfix(16)  OutScaling=2^0  OutDataTypeStr=uint32
  Gain2 : Gain  Gain=-1  ParameterDataType=sfix(16)  ParameterScaling=2^0  OutDataType=sfix(16)  OutScaling=2^0
  Interpolation Using Prelookup : Interpolation_n-D  NumberOfTableDimensions=4  Table=Aero.dC6_spo.data  NumSelectionDims=1  OutDataType=sfix(16)  OutScaling=2^0
  Interpolation Using Prelookup1 : Interpolation_n-D  NumberOfTableDimensions=4  Table=Aero.dC6_spo.data  NumSelectionDims=1  OutDataType=sfix(16)  OutScaling=2^0
  Negate Lateral : Gain  Gain=[1 -1 1 -1 1 -1]  ParameterDataType=sfix(16)  ParameterScaling=2^0  OutDataType=sfix(16)  OutScaling=2^0
  Prelookup1 : PreLookup  BreakpointsData=Aero.dC6_spo.alpha  IndexSearchMethod=Linear search  BeginIndexSearchUsingPreviousIndexResult=on  ProcessOutOfRangeInput=Linear extrapolation  IndexDataType=sfix(16)  FractionDataType=sfix(16)  FractionScaling=2^0
  Prelookup2 : PreLookup  BreakpointsData=Aero.dC6_spo.beta  IndexSearchMethod=Linear search  BeginIndexSearchUsingPreviousIndexResult=on  ProcessOutOfRangeInput=Linear extrapolation  IndexDataType=sfix(16)  FractionDataType=sfix(16)  FractionScaling=2^0
  Prelookup3 : PreLookup  BreakpointsData=Aero.dC6_spo.spo  IndexSearchMethod=Linear search  BeginIndexSearchUsingPreviousIndexResult=on  ProcessOutOfRangeInput=Linear extrapolation  IndexDataType=sfix(16)  FractionDataType=sfix(16)  FractionScaling=2^0
  Prelookup4 : PreLookup  BreakpointsData=Aero.dC6_spo.beta  IndexSearchMethod=Linear search  BeginIndexSearchUsingPreviousIndexResult=on  ProcessOutOfRangeInput=Linear extrapolation  IndexDataType=sfix(16)  FractionDataType=sfix(16)  FractionScaling=2^0
  Prelookup5 : PreLookup  BreakpointsData=Aero.dC6_spo.spo  IndexSearchMethod=Linear search  BeginIndexSearchUsingPreviousIndexResult=on  ProcessOutOfRangeInput=Linear extrapolation  IndexDataType=sfix(16)  FractionDataType=sfix(16)  FractionScaling=2^0
  Left : Outport  OutDataType=sfix(16)  OutScaling=2^0
  Right : Outport  Port=2  OutDataType=sfix(16)  OutScaling=2^0
  wires:
  Gain2/1 -> Prelookup2/1
  Negate Lateral/1 -> Left/1
  Interpolation Using Prelookup1/1 -> Right/1
  SPLRIB/1 -> Prelookup5/1
  beta/1 -> Gain2/1, Prelookup4/1
  alpha/1 -> Prelookup1/1
  SPLLIB/1 -> Prelookup3/1
  Prelookup1/1 -> Interpolation Using Prelookup/1, Interpolation Using Prelookup1/1
  Prelookup1/2 -> Interpolation Using Prelookup/2, Interpolation Using Prelookup1/2
  Prelookup2/1 -> Interpolation Using Prelookup/3
  Prelookup2/2 -> Interpolation Using Prelookup/4
  Prelookup3/1 -> Interpolation Using Prelookup/5
  Prelookup3/2 -> Interpolation Using Prelookup/6
  Constant3/1 -> Interpolation Using Prelookup/7
  Prelookup4/1 -> Interpolation Using Prelookup1/3
  Prelookup4/2 -> Interpolation Using Prelookup1/4
  Prelookup5/1 -> Interpolation Using Prelookup1/5
  Prelookup5/2 -> Interpolation Using Prelookup1/6
  Constant1/1 -> Interpolation Using Prelookup1/7
  Interpolation Using Prelookup/1 -> Negate Lateral/1

== system GTM_aerolib/Dynamic Derviatives/Forced Oscillation with Damage Increments/Damage Effects-Increments ==
  alpha : Inport  OutDataType=sfix(16)  OutScaling=2^0
  pqr : Inport  Port=2  OutDataType=sfix(16)  OutScaling=2^0
  DamageCase : Inport  Port=3  OutDataType=sfix(16)  OutScaling=2^0
  CY derivative increment due to rates : simulink_need_slupdate/Interpolation (n-D) using PreLookup  numDimsPopupSelect=3  explicitNumDims=2  table=squeeze(Aero.dC6_damage.ddinc.data(:,:,:,2))  interpMethod=Linear  extrapMethod=Linear  rangeErrorMode=None  NumSelectionDims=2
  Constant : Constant  Value=uint32(1)  OutDataType=sfix(16)  OutScaling=2^0
  Constant1 : Constant  Value=[0:2]  OutDataTypeMode=uint32  OutDataType=sfix(16)  OutScaling=2^0  OutDataTypeStr=uint32
  Data Type Conversion : DataTypeConversion  OutDataTypeMode=uint32  OutDataType=sfix(16)  OutScaling=2^0  OutDataTypeStr=uint32
  PreLookup Index Search : simulink_need_slupdate/PreLookup Index Search  bpData=Aero.dC6_damage.ddinc.alpha  searchMode=Binary Search  cacheBpFlag=on  outputFlag=off  IndexDataType=uint32  extrapMode=Linear Extrapolation  rangeErrorMode=None
  Product : Product  OutDataType=sfix(16)  OutScaling=2^0  RndMeth=Zero
  Subtract : Sum  Inputs=+-  OutDataType=sfix(16)  OutScaling=2^-10
  Sum of Elements : Sum  Inputs=+  OutDataType=sfix(16)  OutScaling=2^-10
  Increment : Outport  OutDataType=sfix(16)  OutScaling=2^0
  wires:
  Sum of Elements/1 -> Increment/1
  Product/1 -> Sum of Elements/1
  pqr/1 -> Product/2
  CY derivative increment due to rates/1 -> Product/1
  alpha/1 -> PreLookup Index Search/1
  DamageCase/1 -> Data Type Conversion/1
  PreLookup Index Search/1 -> CY derivative increment due to rates/1
  Constant1/1 -> CY derivative increment due to rates/3
  Constant/1 -> Subtract/2
  Data Type Conversion/1 -> Subtract/1
  Subtract/1 -> CY derivative increment due to rates/2

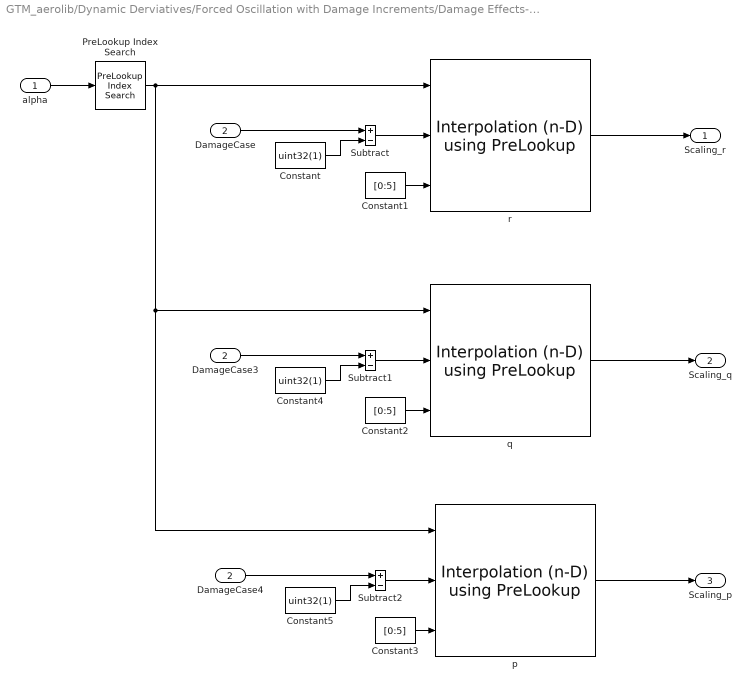
== system GTM_aerolib/Dynamic Derviatives/Forced Oscillation with Damage Increments/Damage Effects-Scaling ==
  alpha : Inport  OutDataType=sfix(16)  OutScaling=2^0
  DamageCase : Inport  Port=2  OutDataType=sfix(16)  OutScaling=2^0
  Constant : Constant  Value=uint32(1)  OutDataType=sfix(16)  OutScaling=2^0
  Constant1 : Constant  Value=[0:5]  OutDataTypeMode=uint32  OutDataType=sfix(16)  OutScaling=2^0  OutDataTypeStr=uint32
  Constant2 : Constant  Value=[0:5]  OutDataTypeMode=uint32  OutDataType=sfix(16)  OutScaling=2^0  OutDataTypeStr=uint32
  Constant3 : Constant  Value=[0:5]  OutDataTypeMode=uint32  OutDataType=sfix(16)  OutScaling=2^0  OutDataTypeStr=uint32
  Constant4 : Constant  Value=uint32(1)  OutDataType=sfix(16)  OutScaling=2^0
  Constant5 : Constant  Value=uint32(1)  OutDataType=sfix(16)  OutScaling=2^0
  DamageCase3 : InportShadow  Port=2  OutDataType=sfix(16)  OutScaling=2^0  LatchByCopyingInsideSignal=off
  DamageCase4 : InportShadow  Port=2  OutDataType=sfix(16)  OutScaling=2^0  LatchByCopyingInsideSignal=off
  PreLookup Index Search : simulink_need_slupdate/PreLookup Index Search  bpData=Aero.dC6_damage.ddscale.alpha  searchMode=Binary Search  cacheBpFlag=on  outputFlag=off  IndexDataType=uint32  extrapMode=Linear Extrapolation  rangeErrorMode=None
  Subtract : Sum  Inputs=+-  OutDataType=sfix(16)  OutScaling=2^-10
  Subtract1 : Sum  Inputs=+-  OutDataType=sfix(16)  OutScaling=2^-10
  Subtract2 : Sum  Inputs=+-  OutDataType=sfix(16)  OutScaling=2^-10
  p : simulink_need_slupdate/Interpolation (n-D) using PreLookup  numDimsPopupSelect=3  explicitNumDims=2  table=squeeze(Aero.dC6_damage.ddscale.data(:,:,1,:))  interpMethod=Linear  extrapMethod=None - Clip  rangeErrorMode=None  NumSelectionDims=2
  q : simulink_need_slupdate/Interpolation (n-D) using PreLookup  numDimsPopupSelect=3  explicitNumDims=2  table=squeeze(Aero.dC6_damage.ddscale.data(:,:,2,:))  interpMethod=Linear  extrapMethod=None - Clip  rangeErrorMode=None  NumSelectionDims=2
  r : simulink_need_slupdate/Interpolation (n-D) using PreLookup  numDimsPopupSelect=3  explicitNumDims=2  table=squeeze(Aero.dC6_damage.ddscale.data(:,:,3,:))  interpMethod=Linear  extrapMethod=None - Clip  rangeErrorMode=None  NumSelectionDims=2
  Scaling_r : Outport  OutDataType=sfix(16)  OutScaling=2^0
  Scaling_q : Outport  Port=2  OutDataType=sfix(16)  OutScaling=2^0
  Scaling_p : Outport  Port=3  OutDataType=sfix(16)  OutScaling=2^0
  wires:
  Constant3/1 -> p/3
  Constant2/1 -> q/3
  Constant1/1 -> r/3
  p/1 -> Scaling_p/1
  q/1 -> Scaling_q/1
  PreLookup Index Search/1 -> p/1, q/1, r/1
  r/1 -> Scaling_r/1
  alpha/1 -> PreLookup Index Search/1
  Constant/1 -> Subtract/2
  Subtract/1 -> r/2
  DamageCase/1 -> Subtract/1
  Constant4/1 -> Subtract1/2
  Constant5/1 -> Subtract2/2
  Subtract1/1 -> q/2
  DamageCase3/1 -> Subtract1/1
  Subtract2/1 -> p/2
  DamageCase4/1 -> Subtract2/1

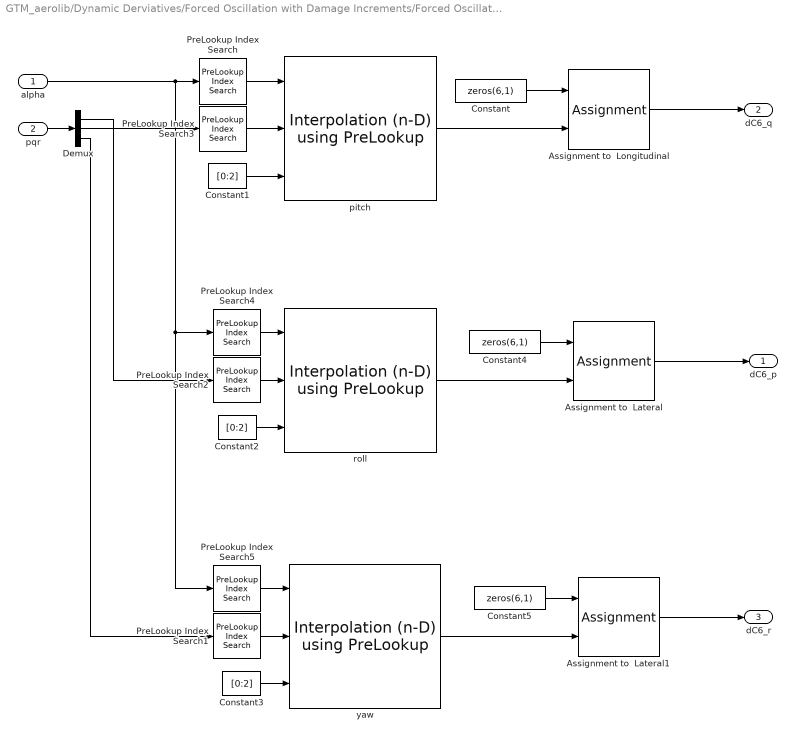
== system GTM_aerolib/Dynamic Derviatives/Forced Oscillation with Damage Increments/Forced Oscillation ==
  alpha : Inport  OutDataType=sfix(16)  OutScaling=2^0
  pqr : Inport  Port=2  OutDataType=sfix(16)  OutScaling=2^0
  Assignment to  Lateral : Assignment  IndexMode=Zero-based  IndexOptions=Index vector (dialog)  Indices=[1 3 5]  OutputSizes=[1 1]
  Assignment to  Lateral1 : Assignment  IndexMode=Zero-based  IndexOptions=Index vector (dialog)  Indices=[1 3 5]  OutputSizes=[1 1]
  Assignment to  Longitudinal : Assignment  IndexMode=Zero-based  IndexOptions=Index vector (dialog)  Indices=[0 2 4]  OutputSizes=[1 1]
  Constant : Constant  Value=zeros(6,1)  OutDataType=sfix(16)  OutScaling=2^0
  Constant1 : Constant  Value=[0:2]  OutDataTypeMode=uint32  OutDataType=sfix(16)  OutScaling=2^0  OutDataTypeStr=uint32
  Constant2 : Constant  Value=[0:2]  OutDataTypeMode=uint32  OutDataType=sfix(16)  OutScaling=2^0  OutDataTypeStr=uint32
  Constant3 : Constant  Value=[0:2]  OutDataTypeMode=uint32  OutDataType=sfix(16)  OutScaling=2^0  OutDataTypeStr=uint32
  Constant4 : Constant  Value=zeros(6,1)  OutDataType=sfix(16)  OutScaling=2^0
  Constant5 : Constant  Value=zeros(6,1)  OutDataType=sfix(16)  OutScaling=2^0
  Demux : Demux  Outputs=3
  PreLookup Index Search : simulink_need_slupdate/PreLookup Index Search  bpData=Aero.dC3_q.alpha  searchMode=Binary Search  cacheBpFlag=on  outputFlag=off  IndexDataType=uint32  extrapMode=Linear Extrapolation  rangeErrorMode=None
  PreLookup Index Search1 : simulink_need_slupdate/PreLookup Index Search  bpData=Aero.dC3_r.rhat  searchMode=Binary Search  cacheBpFlag=on  outputFlag=off  IndexDataType=uint32  extrapMode=Linear Extrapolation  rangeErrorMode=None
  PreLookup Index Search2 : simulink_need_slupdate/PreLookup Index Search  bpData=Aero.dC3_p.phat  searchMode=Binary Search  cacheBpFlag=on  outputFlag=off  IndexDataType=uint32  extrapMode=Linear Extrapolation  rangeErrorMode=None
  PreLookup Index Search3 : simulink_need_slupdate/PreLookup Index Search  bpData=Aero.dC3_q.qhat  searchMode=Binary Search  cacheBpFlag=on  outputFlag=off  IndexDataType=uint32  extrapMode=Linear Extrapolation  rangeErrorMode=None
  PreLookup Index Search4 : simulink_need_slupdate/PreLookup Index Search  bpData=Aero.dC3_p.alpha  searchMode=Binary Search  cacheBpFlag=on  outputFlag=off  IndexDataType=uint32  extrapMode=Linear Extrapolation  rangeErrorMode=None
  PreLookup Index Search5 : simulink_need_slupdate/PreLookup Index Search  bpData=Aero.dC3_r.alpha  searchMode=Binary Search  cacheBpFlag=on  outputFlag=off  IndexDataType=uint32  extrapMode=Linear Extrapolation  rangeErrorMode=None
  pitch : simulink_need_slupdate/Interpolation (n-D) using PreLookup  numDimsPopupSelect=3  explicitNumDims=2  table=Aero.dC3_q.data  interpMethod=Linear  extrapMethod=None - Clip  rangeErrorMode=None  NumSelectionDims=1
  roll : simulink_need_slupdate/Interpolation (n-D) using PreLookup  numDimsPopupSelect=3  explicitNumDims=2  table=Aero.dC3_p.data  interpMethod=Linear  extrapMethod=None - Clip  rangeErrorMode=None  NumSelectionDims=1
  yaw : simulink_need_slupdate/Interpolation (n-D) using PreLookup  numDimsPopupSelect=3  explicitNumDims=2  table=Aero.dC3_r.data  interpMethod=Linear  extrapMethod=None - Clip  rangeErrorMode=None  NumSelectionDims=1
  dC6_p : Outport  OutDataType=sfix(16)  OutScaling=2^0
  dC6_q : Outport  Port=2  OutDataType=sfix(16)  OutScaling=2^0
  dC6_r : Outport  Port=3  OutDataType=sfix(16)  OutScaling=2^0
  wires:
  PreLookup Index Search5/1 -> yaw/1
  PreLookup Index Search4/1 -> roll/1
  PreLookup Index Search/1 -> pitch/1
  Assignment to  Longitudinal/1 -> dC6_q/1
  Assignment to  Lateral1/1 -> dC6_r/1
  Assignment to  Lateral/1 -> dC6_p/1
  PreLookup Index Search3/1 -> pitch/2
  PreLookup Index Search2/1 -> roll/2
  PreLookup Index Search1/1 -> yaw/2
  yaw/1 -> Assignment to  Lateral1/2
  Constant5/1 -> Assignment to  Lateral1/1
  Constant4/1 -> Assignment to  Lateral/1
  roll/1 -> Assignment to  Lateral/2
  pitch/1 -> Assignment to  Longitudinal/2
  Constant/1 -> Assignment to  Longitudinal/1
  Constant3/1 -> yaw/3
  Constant2/1 -> roll/3
  Demux/3 -> PreLookup Index Search1/1
  Demux/1 -> PreLookup Index Search2/1
  Demux/2 -> PreLookup Index Search3/1
  Constant1/1 -> pitch/3
  pqr/1 -> Demux/1
  alpha/1 -> PreLookup Index Search/1, PreLookup Index Search5/1, PreLookup Index Search4/1

== system GTM_aerolib/Dynamic Derviatives/Forced Oscillation with Damage Increments/Normalize ==
  pqr : Inport  OutDataType=sfix(16)  OutScaling=2^0
  TAS : Inport  Port=2  OutDataType=sfix(16)  OutScaling=2^0
  AC_Params : Inport  Port=3  OutDataType=sfix(16)  OutScaling=2^0
  Bus Selector2 : BusSelector  OutputSignals=B,Cbar,B
  Gain : Gain  Gain=2*(1.689)  ParameterDataType=sfix(16)  ParameterScaling=2^0  OutDataType=sfix(16)  OutScaling=2^0
  Mux : Mux  Inputs=3
  Product3 : Product  Inputs=**/  OutDataType=sfix(16)  OutScaling=2^0  RndMeth=Zero
  Saturation1 : Saturate  UpperLimit=10000  LowerLimit=1
  pqrhat : Outport  OutDataType=sfix(16)  OutScaling=2^0
  wires:
  TAS/1 -> Saturation1/1
  AC_Params/1 -> Bus Selector2/1
  Saturation1/1 -> Gain/1
  pqr/1 -> Product3/1
  Gain/1 -> Product3/3
  Product3/1 -> pqrhat/1
  Bus Selector2/1 -> Mux/1  "<B>"
  Bus Selector2/2 -> Mux/2  "<Cbar>"
  Bus Selector2/3 -> Mux/3  "<B>"
  Mux/1 -> Product3/2
